simulink model "eulerEq"  (R2023b)
settings: Solver=ode4  StartTime=0.0  StopTime=30000  FixedStep=0.01  RelTol=1e-3
values from neighbouring files (symbols this model uses):
  date = [2023, 1, 21, 13, 52, 0]    [main.m]    (also in main_nonLin.m)
  euler0 = [0; 0; 0]    [main.m]    (also in main_nonLin.m)
  w0 = h0./sat.I'    [main.m]    (also in main_nonLin.m)
undefined symbols (not defined in the file or in its folder): airDensity, astroConstants, control, DiscIntNeverNeededParam, ea0, earth, gyroscope, magneticConstants, magnetorquer, magSensor, orbit, physicsConstants, rw, sat, sunSensor
libraries: simulink x21, matrix_library x7, sharedtransform x5, dspindex x5, sharedutil x4, vrlib x3, dspfactors x1, simulink_extras x1
(part 1 of 2)
settings Model: PauseTimes=3000  SnapshotBufferSize=100  SnapshotInterval=1  Creator=tomis  LastModifiedBy=francescoantoniomiccoli
settings SolverCC: AlgebraicLoopSolver=TrustRegion
settings DebuggingCC: UnconnectedInputMsg=warning  UnconnectedOutputMsg=warning  UnconnectedLineMsg=warning
settings ModelReferenceCC: EnableRefExpFcnMdlSchedulingChecks=on

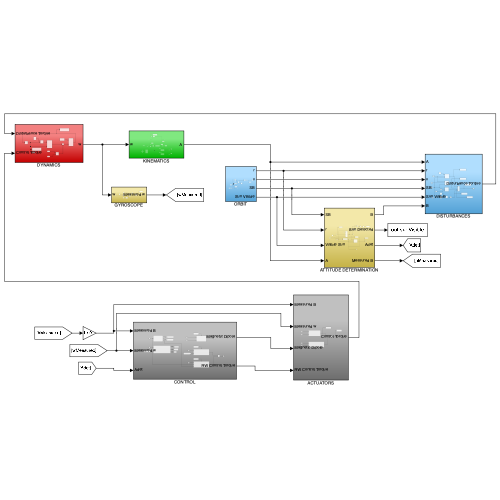
[thumbnail: Simulink's stored preview of the top-level diagram]
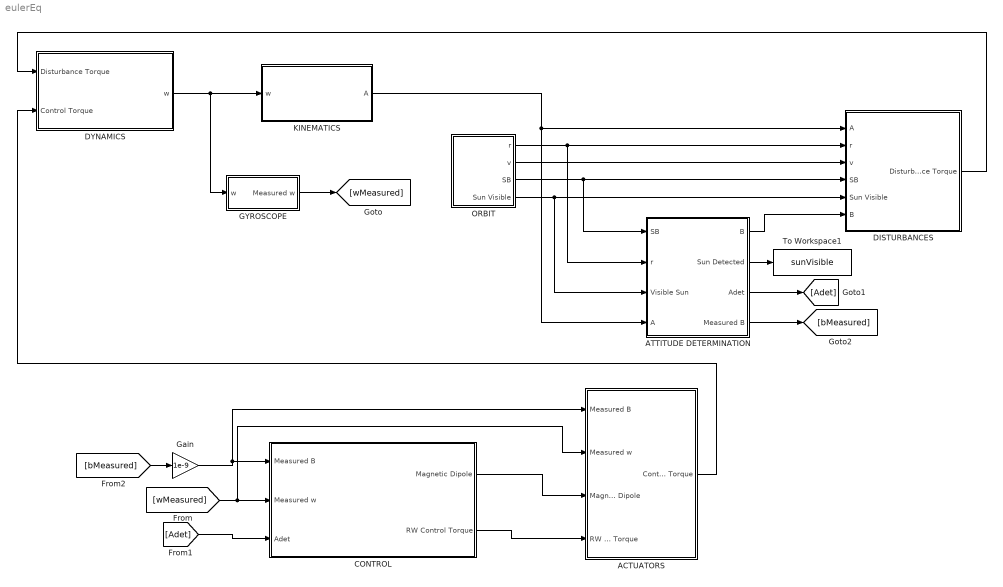
== system eulerEq ==
  ACTUATORS : Subsystem
  ATTITUDE DETERMINATION : Subsystem
  CONTROL : Subsystem
  DISTURBANCES : Subsystem
  DYNAMICS : Subsystem
  GYROSCOPE : Subsystem
  Gain : Gain  Gain=1e-9
  KINEMATICS : Subsystem
  ORBIT : Subsystem
  To Workspace1 : ToWorkspace  VariableName=sunVisible  SampleTime=-1
  wires:
  DYNAMICS/1(w) -> GYROSCOPE/1(w), KINEMATICS/1(w)
  KINEMATICS/1(A) -> DISTURBANCES/1(A), ATTITUDE DETERMINATION/4(A)
  ORBIT/1(r) -> ATTITUDE DETERMINATION/2(r), DISTURBANCES/2(r)
  ORBIT/2(v) -> DISTURBANCES/3(v)
  ORBIT/3(SB) -> ATTITUDE DETERMINATION/1(SB), DISTURBANCES/4(SB)
  ORBIT/4(Sun Visible) -> ATTITUDE DETERMINATION/3(Visible Sun), DISTURBANCES/5(Sun Visible)
  ATTITUDE DETERMINATION/1(B) -> DISTURBANCES/6(B)
  [wMeasured] -> CONTROL/2(Measured w), ACTUATORS/2(Measured w)
  [Adet] -> CONTROL/3(Adet)
  ATTITUDE DETERMINATION/4(Measured B) -> [bMeasured]
  [bMeasured] -> Gain/1
  CONTROL/1(Magnetic Dipole) -> ACTUATORS/3(Magnetic Dipole)
  CONTROL/2(RW Control Torque) -> ACTUATORS/4(RW Control Torque)
  Gain/1 -> CONTROL/1(Measured B), ACTUATORS/1(Measured B)
  DISTURBANCES/1(Disturbance Torque) -> DYNAMICS/1(Disturbance Torque)
  ATTITUDE DETERMINATION/2(Sun Detected) -> To Workspace1/1
  GYROSCOPE/1(Measured w) -> [wMeasured]
  ACTUATORS/1(Control Torque) -> DYNAMICS/2(Control Torque)
  ATTITUDE DETERMINATION/3(Adet) -> [Adet]

== system eulerEq/ACTUATORS ==
  Measured B : Inport
  Measured w : Inport  Port=2
  Magnetic Dipole : Inport  Port=3
  RW Control Torque : Inport  Port=4
  Add : Sum
  MAGNETORQUER : Subsystem
  REACTION WHEELS : Subsystem
  To Workspace : ToWorkspace  VariableName=controlTorque  SampleTime=-1
  To Workspace1 : ToWorkspace  VariableName=magneticTorque  SampleTime=-1
  Control Torque : Outport
  wires:
  Measured B/1 -> MAGNETORQUER/1(Measured B)
  Magnetic Dipole/1 -> MAGNETORQUER/2(Magnetic Dipole)
  MAGNETORQUER/1(Out1) -> To Workspace1/1, Add/1
  Add/1 -> To Workspace/1, Control Torque/1
  Measured w/1 -> REACTION WHEELS/2(Measured w)
  REACTION WHEELS/1(Out1) -> Add/2
  RW Control Torque/1 -> REACTION WHEELS/1(RW Control Torque)

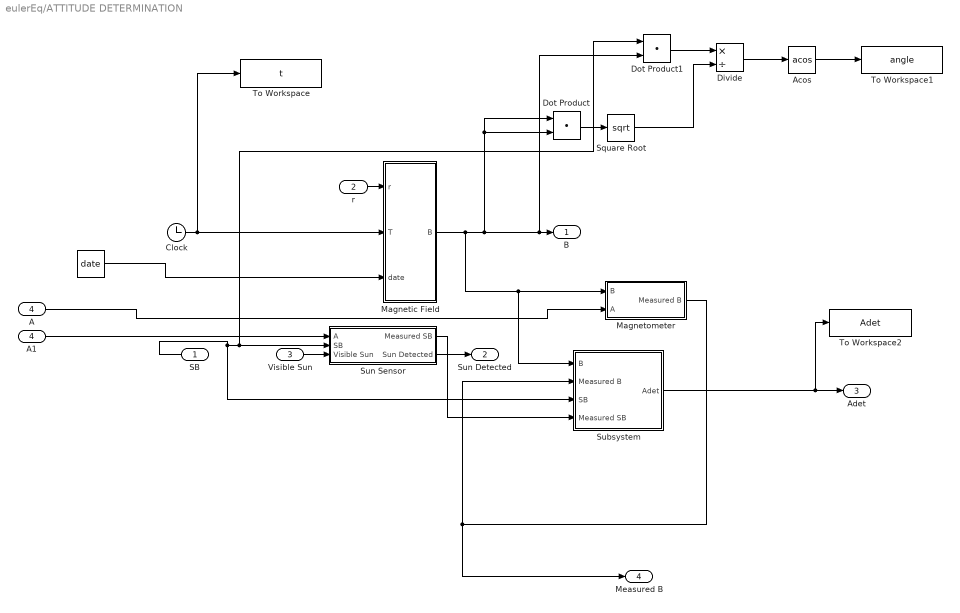
== system eulerEq/ATTITUDE DETERMINATION ==
  SB : Inport
  r : Inport  Port=2
  Visible Sun : Inport  Port=3
  A : Inport  Port=4
  " " : Constant  Value=date  VectorParams1D=off
  A1 : InportShadow  Port=4
  Acos : Trigonometry  Operator=acos
  Clock : Clock
  Divide : Product  Inputs=*/
  Dot Product : DotProduct  OutDataTypeStr=Inherit: Inherit via internal rule
  Dot Product1 : DotProduct  OutDataTypeStr=Inherit: Inherit via internal rule
  Magnetic Field : Subsystem
  Magnetometer : Subsystem
  Square Root : Sqrt
  Subsystem : Subsystem
  Sun Sensor : Subsystem
  To Workspace : ToWorkspace  VariableName=t  SampleTime=-1
  To Workspace1 : ToWorkspace  VariableName=angle  SampleTime=-1
  To Workspace2 : ToWorkspace  VariableName=Adet  SampleTime=-1
  B : Outport
  Sun Detected : Outport  Port=2
  Adet : Outport  Port=3
  Measured B : Outport  Port=4
  wires:
  Sun Sensor/2(Sun Detected) -> Sun Detected/1
  r/1 -> Magnetic Field/1(r)
  " "/1 -> Magnetic Field/3(date)
  Magnetic Field/1(B) -> Dot Product1/2, B/1, Dot Product/1, Dot Product/2, Subsystem/1(B), Magnetometer/1(B)
  Clock/1 -> To Workspace/1, Magnetic Field/2(T)
  Magnetometer/1(Measured B) -> Measured B/1, Subsystem/2(Measured B)
  A1/1 -> Sun Sensor/1(A)
  Subsystem/1(Adet) -> To Workspace2/1, Adet/1
  A/1 -> Magnetometer/2(A)
  Visible Sun/1 -> Sun Sensor/3(Visible Sun)
  SB/1 -> Subsystem/3(SB), Dot Product1/1, Sun Sensor/2(SB)
  Dot Product/1 -> Square Root/1
  Dot Product1/1 -> Divide/1
  Square Root/1 -> Divide/2
  Divide/1 -> Acos/1
  Acos/1 -> To Workspace1/1
  Sun Sensor/1(Measured SB) -> Subsystem/4(Measured SB)

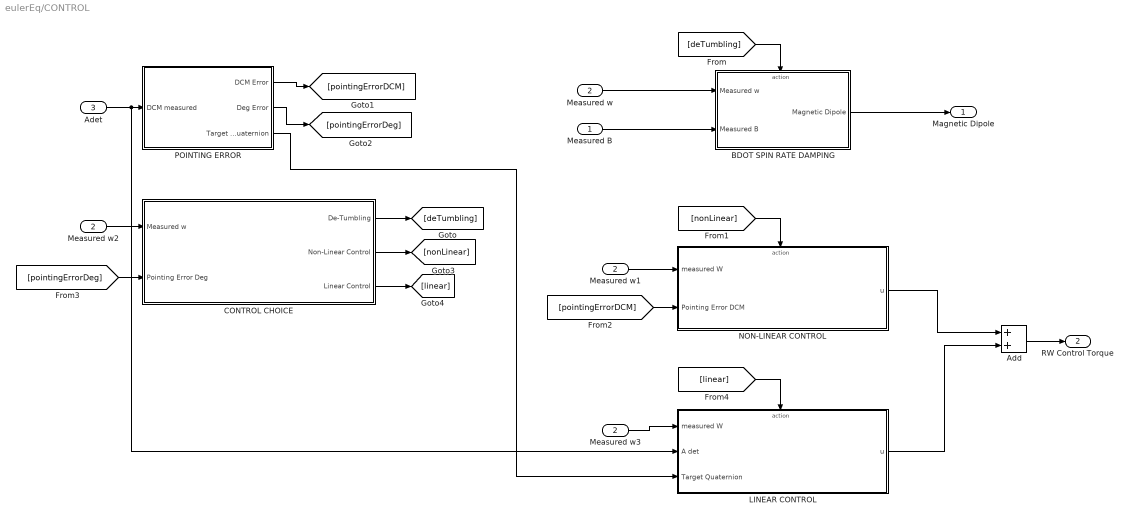
== system eulerEq/CONTROL ==
  Measured B : Inport
  Measured w : Inport  Port=2
  Adet : Inport  Port=3
  Add : Sum
  "BDOT SPIN RATE DAMPING " : Subsystem
  CONTROL CHOICE : Subsystem
  LINEAR CONTROL : Subsystem
  Measured w1 : InportShadow  Port=2
  Measured w2 : InportShadow  Port=2
  Measured w3 : InportShadow  Port=2
  NON-LINEAR CONTROL : Subsystem
  POINTING ERROR : Subsystem
  Magnetic Dipole : Outport
  RW Control Torque : Outport  Port=2
  wires:
  Measured B/1 -> "BDOT SPIN RATE DAMPING "/2(Measured B)
  [linear] -> LINEAR CONTROL/Action
  [nonLinear] -> NON-LINEAR CONTROL/Action
  Measured w2/1 -> CONTROL CHOICE/1(Measured w)
  CONTROL CHOICE/3(Linear Control) -> [linear]
  Add/1 -> RW Control Torque/1
  [pointingErrorDCM] -> NON-LINEAR CONTROL/2(Pointing Error DCM)
  NON-LINEAR CONTROL/1(u) -> Add/1
  Measured w1/1 -> NON-LINEAR CONTROL/1(measured W)
  Measured w/1 -> "BDOT SPIN RATE DAMPING "/1(Measured w)
  [deTumbling] -> "BDOT SPIN RATE DAMPING "/Action
  CONTROL CHOICE/1(De-Tumbling) -> [deTumbling]
  Adet/1 -> LINEAR CONTROL/2(A det), POINTING ERROR/1(DCM measured)
  POINTING ERROR/1(DCM Error) -> [pointingErrorDCM]
  POINTING ERROR/2(Deg Error) -> [pointingErrorDeg]
  [pointingErrorDeg] -> CONTROL CHOICE/2("Pointing Error Deg ")
  LINEAR CONTROL/1(u) -> Add/2
  "BDOT SPIN RATE DAMPING "/1(Magnetic Dipole) -> Magnetic Dipole/1
  CONTROL CHOICE/2(Non-Linear Control) -> [nonLinear]
  Measured w3/1 -> LINEAR CONTROL/1(measured W)
  POINTING ERROR/3(Target Quaternion) -> LINEAR CONTROL/3(Target Quaternion)

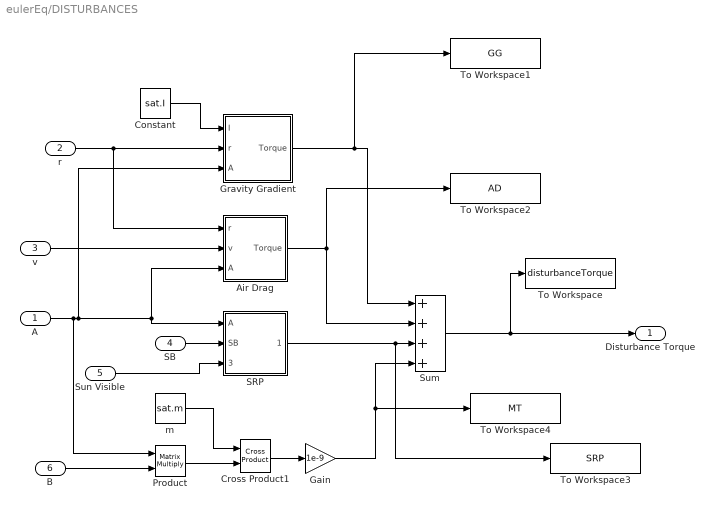
== system eulerEq/DISTURBANCES ==
  A : Inport
  r : Inport  Port=2
  v : Inport  Port=3
  SB : Inport  Port=4
  Sun Visible : Inport  Port=5
  B : Inport  Port=6
  Air Drag : Subsystem
  Constant : Constant  Value=sat.I
  Cross Product1 : vrlib/Utilities/Cross Product
  Gain : Gain  Gain=1e-9
  Gravity Gradient : Subsystem
  Product : Product  Multiplication=Matrix(*)
  SRP : Subsystem
  Sum : Sum  Inputs=++++
  To Workspace : ToWorkspace  VariableName=disturbanceTorque  SampleTime=-1
  To Workspace1 : ToWorkspace  VariableName=GG  SampleTime=-1
  To Workspace2 : ToWorkspace  VariableName=AD  SampleTime=-1
  To Workspace3 : ToWorkspace  VariableName=SRP  SampleTime=-1
  To Workspace4 : ToWorkspace  VariableName=MT  SampleTime=-1
  m : Constant  Value=sat.m
  Disturbance Torque : Outport
  wires:
  A/1 -> Product/1, Gravity Gradient/3(A), Air Drag/3(A), SRP/1(A)
  Sum/1 -> To Workspace/1, Disturbance Torque/1
  Constant/1 -> Gravity Gradient/1(I)
  r/1 -> Air Drag/1(r), Gravity Gradient/2(r)
  v/1 -> Air Drag/2(v)
  SB/1 -> SRP/2(SB)
  m/1 -> Cross Product1/1
  Cross Product1/1 -> Gain/1
  Sun Visible/1 -> SRP/3(Sun Visible)
  Product/1 -> Cross Product1/2
  B/1 -> Product/2
  Gravity Gradient/1(Torque) -> To Workspace1/1, Sum/1
  Air Drag/1(Torque) -> To Workspace2/1, Sum/2
  SRP/1(Torque) -> To Workspace3/1, Sum/3
  Gain/1 -> Sum/4, To Workspace4/1

== system eulerEq/DYNAMICS ==
  Disturbance Torque : Inport
  Control Torque : Inport  Port=2
  Add : Sum
  Constant : Constant  Value=diag(sat.I)
  Constant1 : Constant  Value=inv(diag(sat.I))
  Cross Product : matrix_library/Cross Product
  Integrator : Integrator  InitialCondition=w0
  Product : Product  Multiplication=Matrix(*)
  Product2 : Product  Multiplication=Matrix(*)
  Sum : Sum  Inputs=|++
  To Workspace : ToWorkspace  VariableName=w  SampleTime=-1
  To Workspace1 : ToWorkspace  VariableName=dw  SampleTime=-1
  w : Outport
  wires:
  Disturbance Torque/1 -> Add/1
  Control Torque/1 -> Add/2
  Constant1/1 -> Product/1
  Product/1 -> To Workspace1/1, Integrator/1
  Constant/1 -> Product2/1
  Integrator/1 -> w/1, To Workspace/1, Cross Product/2, Product2/2
  Product2/1 -> Cross Product/1
  Cross Product/1 -> Sum/1
  Add/1 -> Sum/2
  Sum/1 -> Product/2

== system eulerEq/GYROSCOPE ==
  w : Inport
  ARW : RandomNumber  Variance=gyroscope.stdDeviation^2  Seed=12984537  SampleTime=gyroscope.Ts  VectorParams1D=off
  Add : Sum  Inputs=+++
  Discrete-Time Integrator : DiscreteIntegrator  IntegratorMethod=Integration: Trapezoidal  SampleTime=gyroscope.Ts  ICPrevOutput=DiscIntNeverNeededParam  ICPrevScaledInput=DiscIntNeverNeededParam
  MatrixMultiply : Product  Multiplication=Matrix(*)
  MatrixMultiply1 : Product  Multiplication=Matrix(*)
  RRW : RandomNumber  Variance=gyroscope.biasStability^2  Seed=34654365  SampleTime=gyroscope.Ts  VectorParams1D=off
  Rotation B-S : Constant  Value=eye(3)
  Rotation S-B : Constant  Value=eye(3)
  To Workspace5 : ToWorkspace  VariableName=wdet  SampleTime=-1
  Measured w : Outport
  wires:
  Add/1 -> MatrixMultiply1/2
  Rotation S-B/1 -> MatrixMultiply1/1
  Discrete-Time Integrator/1 -> Add/3
  MatrixMultiply/1 -> Add/2
  w/1 -> MatrixMultiply/2
  Rotation B-S/1 -> MatrixMultiply/1
  ARW/1 -> Add/1
  RRW/1 -> Discrete-Time Integrator/1
  MatrixMultiply1/1 -> To Workspace5/1, Measured w/1

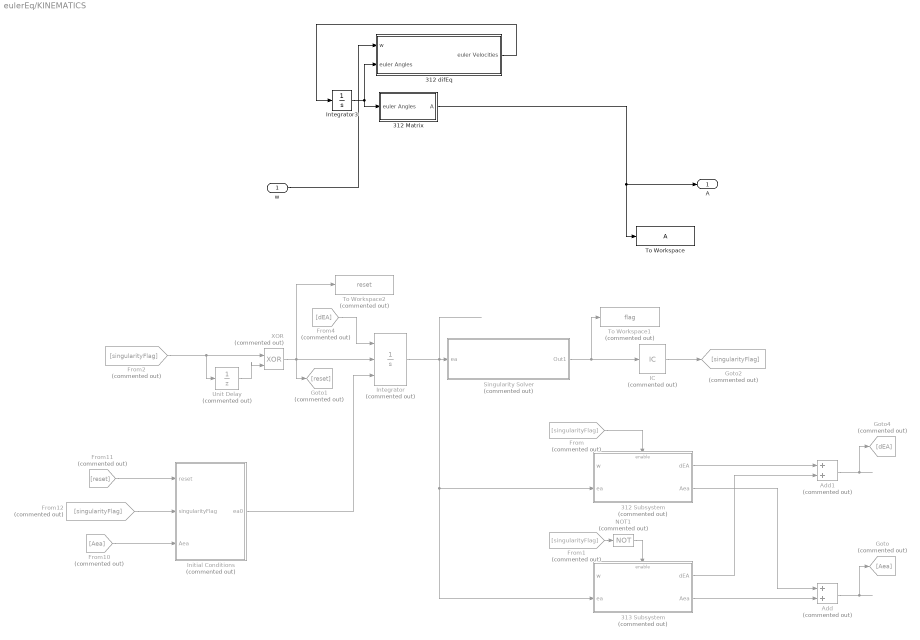
== system eulerEq/KINEMATICS ==
  w : Inport
  312 Matrix : Subsystem
  312 Subsystem : Subsystem  Commented=on  TreatAsAtomicUnit=on
  312 difEq : Subsystem
  313 Subsystem : Subsystem  Commented=on  TreatAsAtomicUnit=on
  Add : Sum  Commented=on
  Add1 : Sum  Commented=on
  From{,1..2,12} (4 alike) : From  Commented=on  GotoTag=singularityFlag
  From10 : From  Commented=on  GotoTag=Aea
  From11 : From  Commented=on  GotoTag=reset
  From4 : From  Commented=on  GotoTag=dEA
  Goto : Goto  Commented=on  GotoTag=Aea
  Goto1 : Goto  Commented=on  GotoTag=reset
  Goto2 : Goto  Commented=on  GotoTag=singularityFlag
  Goto4 : Goto  Commented=on  GotoTag=dEA
  IC : InitialCondition  Commented=on
  Initial Conditions : Subsystem  Commented=on
  Integrator : Integrator  Commented=on  ExternalReset=rising  InitialConditionSource=external
  Integrator3 : Integrator  InitialCondition=euler0
  NOT1 : Logic  Commented=on  Operator=NOT  AllPortsSameDT=off  OutDataTypeStr=boolean
  Singularity Solver : Subsystem  Commented=on
  To Workspace : ToWorkspace  VariableName=A  SampleTime=-1
  To Workspace1 : ToWorkspace  Commented=on  VariableName=flag  SampleTime=-1
  To Workspace2 : ToWorkspace  Commented=on  VariableName=reset  SampleTime=-1
  Unit Delay : UnitDelay  Commented=on  InitialCondition=1  SampleTime=-1  HasFrameUpgradeWarning=on
  XOR : Logic  Commented=on  Operator=XOR  IconShape=distinctive  AllPortsSameDT=off  OutDataTypeStr=boolean
  A : Outport
  wires:
  312 difEq/1(euler Velocities) -> Integrator3/1
  Integrator3/1 -> 312 Matrix/1(euler Angles), 312 difEq/2(euler Angles)
  w/1 -> 312 difEq/1(w)
  312 Matrix/1(A) -> To Workspace/1, A/1
  Singularity Solver/1(Out1) -> IC/1, To Workspace1/1
  312 Subsystem/2(Aea) -> Add/1
  313 Subsystem/1(dEA) -> Add1/2
  312 Subsystem/1(dEA) -> Add1/1
  Integrator/1 -> 313 Subsystem/2(ea), 312 Subsystem/2(ea), Singularity Solver/1(ea)
  Add1/1 -> Goto4/1
  IC/1 -> Goto2/1
  From10/1 -> Initial Conditions/3(Aea)
  From1/1 -> NOT1/1
  XOR/1 -> To Workspace2/1, Integrator/2, Goto1/1
  313 Subsystem/2(Aea) -> Add/2
  From4/1 -> Integrator/1
  From12/1 -> Initial Conditions/2(singularityFlag)
  From2/1 -> Unit Delay/1, XOR/1
  From11/1 -> Initial Conditions/1(reset)
  From/1 -> 312 Subsystem/Enable
  Unit Delay/1 -> XOR/2
  Add/1 -> Goto/1
  NOT1/1 -> 313 Subsystem/Enable
  Initial Conditions/1(ea0) -> Integrator/3

== system eulerEq/ORBIT ==
  Cross Product : matrix_library/Cross Product
  Cross Product1 : matrix_library/Cross Product
  Earth Orbit : Subsystem
  Gain2 : Gain  Gain=-1
  Matrix Concatenate : Concatenate  NumInputs=3  Mode=Multidimensional array  ConcatenateDimension=2
  Normalize1 : Subsystem
  Normalize2 : Subsystem
  Normalize3 : Subsystem
  Sat Orbit : Subsystem
  Sun Detection : Subsystem
  To Workspace : ToWorkspace  VariableName=DCMTarget  SampleTime=-1
  To Workspace1 : ToWorkspace  VariableName=rorbit  SampleTime=-1
  Transpose : Math  Operator=transpose
  r : Outport
  v : Outport  Port=2
  SB : Outport  Port=3
  Sun Visible : Outport  Port=4
  tag scope: DCMTarget=global
  wires:
  Sat Orbit/1(r) -> Sun Detection/1(r), Normalize2/1(r), To Workspace1/1, r/1
  Earth Orbit/1(r) -> Normalize1/1(r)
  Normalize1/1(Out) -> Gain2/1
  Sat Orbit/2(v) -> Normalize3/1(r), v/1
  Gain2/1 -> Sun Detection/2(SB), SB/1
  Sun Detection/1(Sun Visible) -> Sun Visible/1
  Normalize2/1(Out) -> Cross Product1/2, Matrix Concatenate/3, Cross Product/1
  Normalize3/1(Out) -> Cross Product/2
  Cross Product/1 -> Matrix Concatenate/2, Cross Product1/1
  Cross Product1/1 -> Matrix Concatenate/1
  Matrix Concatenate/1 -> Transpose/1
  Transpose/1 -> To Workspace/1, [DCMTarget]

== system eulerEq/ACTUATORS/MAGNETORQUER ==
  Measured B : Inport
  Magnetic Dipole : Inport  Port=2
  Cross Product : matrix_library/Cross Product
  Saturation : Saturate  UpperLimit=magnetorquer.m  LowerLimit=-magnetorquer.m
  To Workspace : ToWorkspace  VariableName=dipole  SampleTime=-1
  Out1 : Outport
  wires:
  Magnetic Dipole/1 -> Saturation/1
  Measured B/1 -> Cross Product/2
  Cross Product/1 -> Out1/1
  Saturation/1 -> To Workspace/1, Cross Product/1

== system eulerEq/ACTUATORS/REACTION WHEELS ==
  RW Control Torque : Inport
  Measured w : Inport  Port=2
  Add : Sum
  Add1 : Sum
  Constant : Constant  Value=rw.Ainv
  Constant1 : Constant  Value=rw.A
  Cross Product : matrix_library/Cross Product
  Gain : Gain  Gain=-1
  Gain1 : Gain  Gain=-1
  Integrator : Integrator
  Product : Product  Multiplication=Matrix(*)
  Product1 : Product  Multiplication=Matrix(*)
  Product2 : Product  Multiplication=Matrix(*)
  Saturation : Saturate  UpperLimit=rw.dhMax  LowerLimit=-rw.dhMax
  Saturation1 : Saturate  UpperLimit=rw.hMax  LowerLimit=-rw.hMax
  To Workspace : ToWorkspace  VariableName=hr  SampleTime=-1
  To Workspace1 : ToWorkspace  VariableName=dhr  SampleTime=-1
  Out1 : Outport
  wires:
  Constant/1 -> Gain/1
  Gain/1 -> Product/1
  Measured w/1 -> Cross Product/1
  Product1/1 -> Cross Product/2
  Constant1/1 -> Product1/1, Product2/1
  Cross Product/1 -> Add1/1, Add/2
  Add/1 -> Product/2
  RW Control Torque/1 -> Add/1
  Product/1 -> Saturation/1
  Product2/1 -> Add1/2
  Add1/1 -> Gain1/1
  Gain1/1 -> Out1/1
  Integrator/1 -> Saturation1/1
  Saturation/1 -> To Workspace1/1, Integrator/1, Product2/2
  Saturation1/1 -> To Workspace/1, Product1/2

== system eulerEq/ATTITUDE DETERMINATION/Magnetic Field ==
  r : Inport
  T : Inport  Port=2
  date : Inport  Port=3
  MATLAB Function : MATLAB Function  TreatAsAtomicUnit=on
  Transpose : Math  Operator=transpose
  igrfSg : Constant  Value=magneticConstants.igrfSg
  igrfSh : Constant  Value=magneticConstants.igrfSh
  B : Outport
  wires:
  igrfSh/1 -> MATLAB Function/5(igrfSh)
  T/1 -> MATLAB Function/2(T)
  igrfSg/1 -> MATLAB Function/4(igrfSg)
  r/1 -> Transpose/1
  date/1 -> MATLAB Function/3(date)
  Transpose/1 -> MATLAB Function/1(r)
  MATLAB Function/1(B) -> B/1

== system eulerEq/ATTITUDE DETERMINATION/Magnetometer ==
  B : Inport
  A : Inport  Port=2
  Band-Limited White Noise : simulink/Sources/Band-Limited White Noise  Cov=magSensor.noisePower*[1;1;1]  Ts=1/magSensor.sampleRate  seed=[3563456;34634;7567457]  VectorParams1D=off
  Product : Product  Multiplication=Matrix(*)
  Quantizer : Quantizer  QuantizationInterval=magSensor.resolution
  Sum : Sum  Inputs=|++
  Zero-Order Hold : ZeroOrderHold  SampleTime=1/magSensor.sampleRate
  Measured B : Outport
  wires:
  Zero-Order Hold/1 -> Sum/1
  Band-Limited White Noise/1 -> Sum/2
  Sum/1 -> Quantizer/1
  Quantizer/1 -> Measured B/1
  B/1 -> Product/2
  Product/1 -> Zero-Order Hold/1
  A/1 -> Product/1

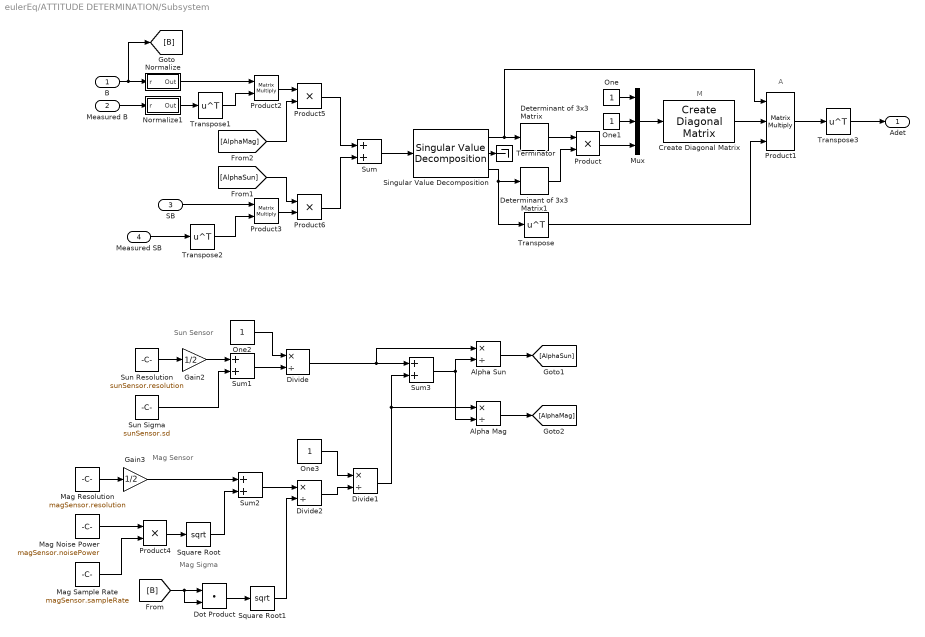
== system eulerEq/ATTITUDE DETERMINATION/Subsystem ==
  note: Mag Sigma
  note: Sun Sensor
  note: A
  note: M
  note: Mag Sensor
  B : Inport
  Measured B : Inport  Port=2
  SB : Inport  Port=3
  Measured SB : Inport  Port=4
  Alpha Mag : Product  Inputs=*/
  Alpha Sun : Product  Inputs=*/
  Create Diagonal Matrix : matrix_library/Create Diagonal Matrix
      settings: LibrarySourceBlock=|
      | simulink/Matrix
      | Operations/Create Diagonal
      | Matrix
  Determinant of 3x3 Matrix : sharedutil/Determinant of 3x3 Matrix  aMode=aMode
      settings: LibrarySourceBlock=|
      | aerolibutil/Determinant of
      | 3x3 Matrix
  Determinant of 3x3 Matrix1 : sharedutil/Determinant of 3x3 Matrix  aMode=aMode
      settings: LibrarySourceBlock=|
      | aerolibutil/Determinant of
      | 3x3 Matrix
  Divide : Product  Inputs=*/
  Divide1 : Product  Inputs=*/
  Divide2 : Product  Inputs=*/
  Dot Product : DotProduct  OutDataTypeStr=Inherit: Inherit via internal rule
  Gain2 : Gain  Gain=1/2
  Gain3 : Gain  Gain=1/2
  Mag Noise Power : Constant  Value=magSensor.noisePower
  Mag Resolution : Constant  Value=magSensor.resolution
  Mag Sample Rate : Constant  Value=magSensor.sampleRate
  Mux : Mux  Inputs=3
  Normalize : Subsystem
  Normalize1 : Subsystem
  One{,1..3} (4 alike) : Constant  OutDataTypeStr=Inherit: Inherit via back propagation
  Product{,4..6} (4 alike) : Product
  Product1 : Product  Inputs=3  Multiplication=Matrix(*)
  Product2 : Product  Multiplication=Matrix(*)
  Product3 : Product  Multiplication=Matrix(*)
  Singular Value Decomposition : dspfactors/Singular Value Decomposition  wantv=on  wanterr=off  SimulateUsing=Interpreted execution
  Square Root : Sqrt
  Square Root1 : Sqrt
  Sum{,1..3} (4 alike) : Sum
  Sun Resolution : Constant  Value=sunSensor.resolution
  Sun Sigma : Constant  Value=sunSensor.sd
  Terminator : Terminator
  Transpose{,1..3} (4 alike) : Math  Operator=transpose
  Adet : Outport
  wires:
  Sum/1 -> Singular Value Decomposition/1
  One/1 -> Mux/1
  Normalize1/1(Out) -> Transpose1/1
  Singular Value Decomposition/1 -> Determinant of 3x3 Matrix/1, Product1/1
  Create Diagonal Matrix/1 -> Product1/2
  Transpose/1 -> Product1/3
  Singular Value Decomposition/3 -> Transpose/1, Determinant of 3x3 Matrix1/1
  One1/1 -> Mux/2
  Transpose2/1 -> Product3/2
  Determinant of 3x3 Matrix/1 -> Product/1
  Measured B/1 -> Normalize1/1(r)
  Singular Value Decomposition/2 -> Terminator/1
  Determinant of 3x3 Matrix1/1 -> Product/2
  Mux/1 -> Create Diagonal Matrix/1
  Product/1 -> Mux/3
  Transpose1/1 -> Product2/2
  Product1/1 -> Transpose3/1
  Normalize/1(Out) -> Product2/1
  B/1 -> [B], Normalize/1(r)
  SB/1 -> Product3/1
  Measured SB/1 -> Transpose2/1
  Sun Resolution/1 -> Gain2/1
  Gain2/1 -> Sum1/1
  Sun Sigma/1 -> Sum1/2
  Sum1/1 -> Divide/2
  One2/1 -> Divide/1
  Mag Noise Power/1 -> Product4/1
  Mag Sample Rate/1 -> Product4/2
  Product4/1 -> Square Root/1
  Mag Resolution/1 -> Gain3/1
  Gain3/1 -> Sum2/1
  Square Root/1 -> Sum2/2
  One3/1 -> Divide1/1
  Divide/1 -> Alpha Sun/1, Sum3/1
  Divide1/1 -> Sum3/2, Alpha Mag/1
  Sum3/1 -> Alpha Mag/2, Alpha Sun/2
  Sum2/1 -> Divide2/1
  Divide2/1 -> Divide1/2
  Product2/1 -> Product5/1
  Product3/1 -> Product6/2
  Alpha Sun/1 -> [AlphaSun]
  Alpha Mag/1 -> [AlphaMag]
  [AlphaSun] -> Product6/1
  [AlphaMag] -> Product5/2
  Product5/1 -> Sum/1
  Product6/1 -> Sum/2
  [B] -> Dot Product/2, Dot Product/1
  Dot Product/1 -> Square Root1/1
  Square Root1/1 -> Divide2/2
  Transpose3/1 -> Adet/1

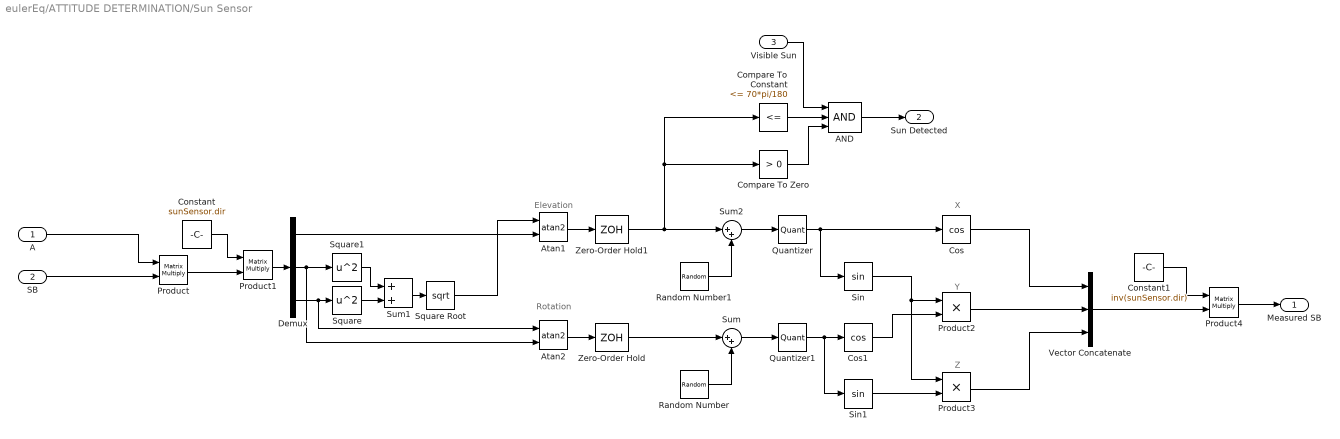
== system eulerEq/ATTITUDE DETERMINATION/Sun Sensor ==
  note: Y
  note: Z
  note: X
  note: Rotation
  note: Elevation
  A : Inport
  SB : Inport  Port=2
  Visible Sun : Inport  Port=3
  AND : Logic  Inputs=3  IconShape=distinctive  AllPortsSameDT=off  OutDataTypeStr=boolean
  Atan1 : Trigonometry  Operator=atan2
  Atan2 : Trigonometry  Operator=atan2
  Compare To Constant : simulink/Logic and Bit Operations/Compare To Constant  relop=<=  const=70*pi/180  OutDataTypeStr=boolean
  Compare To Zero : simulink/Logic and Bit Operations/Compare To Zero  relop=>  OutDataTypeStr=boolean
  Constant : Constant  Value=sunSensor.dir
  Constant1 : Constant  Value=inv(sunSensor.dir)
  Cos : Trigonometry  Operator=cos
  Cos1 : Trigonometry  Operator=cos
  Demux : Demux  Outputs=3
  Product : Product  Multiplication=Matrix(*)
  Product1 : Product  Multiplication=Matrix(*)
  Product2 : Product
  Product3 : Product
  Product4 : Product  Multiplication=Matrix(*)
  Quantizer : Quantizer  QuantizationInterval=sunSensor.resolution
  Quantizer1 : Quantizer  QuantizationInterval=sunSensor.resolution
  Random Number : RandomNumber  Variance=sunSensor.sd^2  Seed=76538356  SampleTime=1/sunSensor.sampleRate
  Random Number1 : RandomNumber  Variance=sunSensor.sd^2  Seed=45746823  SampleTime=1/sunSensor.sampleRate
  Sin : Trigonometry
  Sin1 : Trigonometry
  Square : Math  Operator=square
  Square Root : Sqrt
  Square1 : Math  Operator=square
  Sum : Sum  Inputs=|++
  Sum1 : Sum
  Sum2 : Sum  Inputs=|++
  Vector Concatenate : Concatenate  NumInputs=3  ConcatenateDimension=2
  Zero-Order Hold : ZeroOrderHold  SampleTime=1/sunSensor.sampleRate
  Zero-Order Hold1 : ZeroOrderHold  SampleTime=1/sunSensor.sampleRate
  Measured SB : Outport
  Sun Detected : Outport  Port=2
  wires:
  Cos1/1 -> Product2/2
  Square/1 -> Sum1/2
  Zero-Order Hold/1 -> Sum/1
  Square1/1 -> Sum1/1
  Random Number/1 -> Sum/2
  Sum2/1 -> Quantizer/1
  Product/1 -> Product1/2
  Sin/1 -> Product3/1, Product2/1
  Constant/1 -> Product1/1
  Demux/2 -> Square1/1, Atan2/2
  Demux/3 -> Atan2/1, Square/1
  Sin1/1 -> Product3/2
  Atan2/1 -> Zero-Order Hold/1
  Atan1/1 -> Zero-Order Hold1/1
  Product1/1 -> Demux/1
  Sum1/1 -> Square Root/1
  Quantizer1/1 -> Sin1/1, Cos1/1
  Zero-Order Hold1/1 -> Compare To Zero/1, Compare To Constant/1, Sum2/1
  Product2/1 -> Vector Concatenate/2
  Sum/1 -> Quantizer1/1
  A/1 -> Product/1
  SB/1 -> Product/2
  Product3/1 -> Vector Concatenate/3
  Quantizer/1 -> Sin/1, Cos/1
  Cos/1 -> Vector Concatenate/1
  Vector Concatenate/1 -> Product4/2
  Constant1/1 -> Product4/1
  Product4/1 -> Measured SB/1
  Random Number1/1 -> Sum2/2
  Compare To Constant/1 -> AND/2
  Visible Sun/1 -> AND/1
  AND/1 -> Sun Detected/1
  Compare To Zero/1 -> AND/3
  Demux/1 -> Atan1/2
  Square Root/1 -> Atan1/1

== system eulerEq/CONTROL/BDOT SPIN RATE DAMPING  ==
  Measured w : Inport
  Measured B : Inport  Port=2
  Action Port : ActionPort  ActionPortLabel=else
  CROSS MATRIX : Subsystem
  Constant : Constant  Value=-5e7
  Gain : Gain  Gain=-1
  Product : Product  Multiplication=Matrix(*)
  Product1 : Product
  Magnetic Dipole : Outport  OutputWhenDisabled=reset  InitialOutput=[0;0;0]
  wires:
  Measured w/1 -> CROSS MATRIX/1(Measured w)
  CROSS MATRIX/1(w^) -> Gain/1
  Gain/1 -> Product/1
  Measured B/1 -> Product/2
  Product/1 -> Product1/2  "dB"
  Product1/1 -> Magnetic Dipole/1
  Constant/1 -> Product1/1

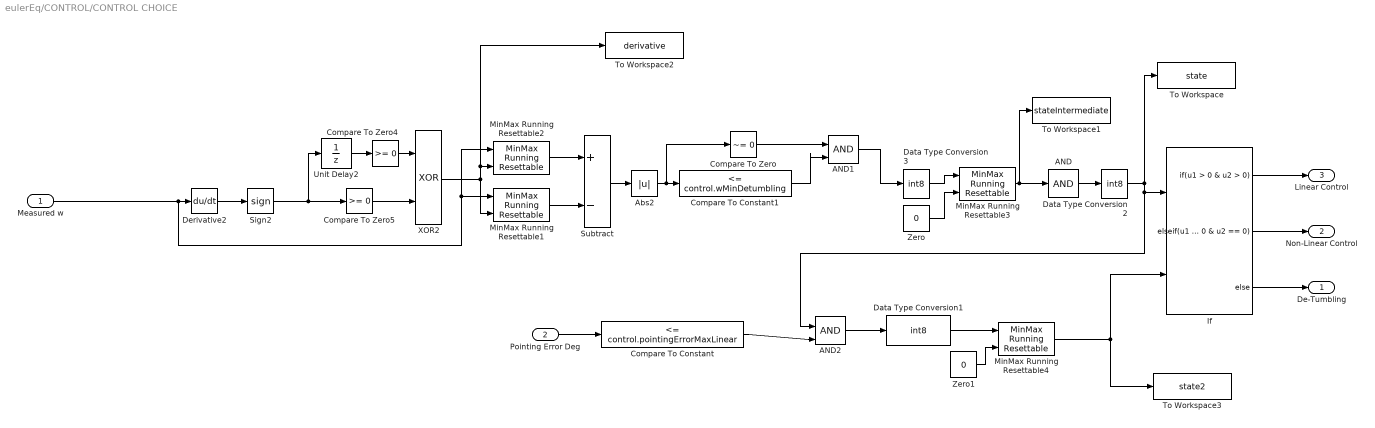
== system eulerEq/CONTROL/CONTROL CHOICE ==
  Measured w : Inport
  "Pointing Error Deg " : Inport  Port=2
  AND : Logic  Inputs=1  IconShape=distinctive  AllPortsSameDT=off  OutDataTypeStr=boolean
  AND1 : Logic  IconShape=distinctive  AllPortsSameDT=off  OutDataTypeStr=boolean
  AND2 : Logic  IconShape=distinctive  AllPortsSameDT=off  OutDataTypeStr=boolean
  Abs2 : Abs  SaturateOnIntegerOverflow=off
  Compare To Constant : simulink/Logic and Bit Operations/Compare To Constant  relop=<=  const=control.pointingErrorMaxLinear  OutDataTypeStr=boolean
  Compare To Constant1 : simulink/Logic and Bit Operations/Compare To Constant  relop=<=  const=control.wMinDetumbling  OutDataTypeStr=boolean
  Compare To Zero : simulink/Logic and Bit Operations/Compare To Zero  relop=~=  OutDataTypeStr=boolean
  Compare To Zero4 : simulink/Logic and Bit Operations/Compare To Zero  relop=>=  OutDataTypeStr=boolean
  Compare To Zero5 : simulink/Logic and Bit Operations/Compare To Zero  relop=>=  OutDataTypeStr=boolean
  Data Type Conversion1 : DataTypeConversion  OutDataTypeStr=int8  SaturateOnIntegerOverflow=off  RndMeth=Floor
  Data Type Conversion2 : DataTypeConversion  OutDataTypeStr=int8  SaturateOnIntegerOverflow=off  RndMeth=Floor
  Data Type Conversion3 : DataTypeConversion  OutDataTypeStr=int8  SaturateOnIntegerOverflow=off  RndMeth=Floor
  Derivative2 : Derivative
  If : If  NumInputs=2  IfExpression=u1 > 0 & u2 > 0  ElseIfExpressions=u1 > 0 & u2 == 0
  MinMax Running Resettable1 : simulink/Math Operations/MinMax Running Resettable  Function=min  vinit=0.0
  MinMax Running Resettable2 : simulink/Math Operations/MinMax Running Resettable  Function=max  vinit=0
  MinMax Running Resettable3 : simulink/Math Operations/MinMax Running Resettable  Function=max  vinit=0
  MinMax Running Resettable4 : simulink/Math Operations/MinMax Running Resettable  Function=max  vinit=0
  Sign2 : Signum
  Subtract : Sum  Inputs=+-
  To Workspace : ToWorkspace  VariableName=state  SampleTime=-1
  To Workspace1 : ToWorkspace  VariableName=stateIntermediate  SampleTime=-1
  To Workspace2 : ToWorkspace  VariableName=derivative  SampleTime=-1
  To Workspace3 : ToWorkspace  VariableName=state2  SampleTime=-1
  Unit Delay2 : UnitDelay  InitialCondition=-1  SampleTime=-1  HasFrameUpgradeWarning=on
  XOR2 : Logic  Operator=XOR  AllPortsSameDT=off  OutDataTypeStr=boolean
  Zero : Constant  Value=0  OutDataTypeStr=Inherit: Inherit via back propagation
  Zero1 : Constant  Value=0  OutDataTypeStr=Inherit: Inherit via back propagation
  De-Tumbling : Outport
  Non-Linear Control : Outport  Port=2
  Linear Control : Outport  Port=3
  wires:
  Derivative2/1 -> Sign2/1
  Sign2/1 -> Unit Delay2/1, Compare To Zero5/1
  Compare To Zero5/1 -> XOR2/2
  Compare To Zero4/1 -> XOR2/1
  Unit Delay2/1 -> Compare To Zero4/1
  "Pointing Error Deg "/1 -> Compare To Constant/1
  If/1 -> Linear Control/1
  If/2 -> Non-Linear Control/1
  If/3 -> De-Tumbling/1
  XOR2/1 -> MinMax Running Resettable2/2, To Workspace2/1, MinMax Running Resettable1/2
  MinMax Running Resettable2/1 -> Subtract/1
  MinMax Running Resettable1/1 -> Subtract/2
  Abs2/1 -> Compare To Zero/1, Compare To Constant1/1
  Subtract/1 -> Abs2/1
  AND/1 -> Data Type Conversion2/1
  Data Type Conversion2/1 -> AND2/1, If/1, To Workspace/1
  MinMax Running Resettable3/1 -> To Workspace1/1, AND/1
  Data Type Conversion3/1 -> MinMax Running Resettable3/1
  Measured w/1 -> Derivative2/1, MinMax Running Resettable2/1, MinMax Running Resettable1/1
  Compare To Constant1/1 -> AND1/2
  AND1/1 -> Data Type Conversion3/1
  Compare To Zero/1 -> AND1/1
  Data Type Conversion1/1 -> MinMax Running Resettable4/1
  MinMax Running Resettable4/1 -> To Workspace3/1, If/2
  Zero/1 -> MinMax Running Resettable3/2
  Zero1/1 -> MinMax Running Resettable4/2
  AND2/1 -> Data Type Conversion1/1
  Compare To Constant/1 -> AND2/2

== system eulerEq/CONTROL/LINEAR CONTROL ==
  measured W : Inport
  A det : Inport  Port=2
  Target Quaternion : Inport  Port=3
  Action Port : ActionPort  ActionPortLabel=if(u1 > 0 & u2 > 0)
  Add : Sum  Inputs=-+
  Constant : Constant  Value=control.K
  Constant1 : Constant  Value=[control.wTarget]
  Direction Cosine Matrix to Quaternions : sharedtransform/Direction Cosine Matrix  to Quaternions  aMode=0  action=None  tolerance=eps(2)
      settings: LibrarySourceBlock=|
      | aerolibtransform2/Direction Cosine Matrix
      | to Quaternions
  Matrix Concatenate : Concatenate  Mode=Multidimensional array
  Product : Product  Multiplication=Matrix(*)
  Vector Concatenate : Concatenate
  u : Outport  OutputWhenDisabled=reset  InitialOutput=[0;0;0]
  wires:
  A det/1 -> Direction Cosine Matrix to Quaternions/1
  measured W/1 -> Vector Concatenate/1
  Constant/1 -> Product/1
  Direction Cosine Matrix to Quaternions/1 -> Vector Concatenate/2
  Vector Concatenate/1 -> Add/1
  Add/1 -> Product/2
  Product/1 -> u/1
  Constant1/1 -> Matrix Concatenate/1
  Target Quaternion/1 -> Matrix Concatenate/2
  Matrix Concatenate/1 -> Add/2

== system eulerEq/CONTROL/NON-LINEAR CONTROL ==
  measured W : Inport
  Pointing Error DCM : Inport  Port=2
  Action Port : ActionPort  ActionPortLabel=elseif(u1 > 0 & u2 == 0)
  Add1 : Sum
  Gain1 : Gain  Gain=-0.4
  Gain3 : Gain  Gain=-0.006
  u : Outport  OutputWhenDisabled=reset  InitialOutput=[0;0;0]
  wires:
  Add1/1 -> u/1
  Gain1/1 -> Add1/1
  measured W/1 -> Gain1/1
  Pointing Error DCM/1 -> Gain3/1
  Gain3/1 -> Add1/2

== system eulerEq/CONTROL/POINTING ERROR ==
  DCM measured : Inport
  Add : Sum  Inputs=+-
  Demux : Demux  Outputs=3
  Demux1 : Demux  Outputs=3
  Direction Cosine Matrix to Quaternions : sharedtransform/Direction Cosine Matrix  to Quaternions  aMode=0  action=None  tolerance=eps(2)
      settings: LibrarySourceBlock=|
      | aerolibtransform2/Direction Cosine Matrix
      | to Quaternions
  Gain : Gain  Gain=-1
  Gain1 : Gain  Gain=-1
  Multiport Selector : dspindex/Multiport Selector  rowsOrCols=Rows  idxCellArray={ 1,2 }  idxErrMode=Clip Index
      settings: LibrarySourceBlock=|
      | dsphdlsupportsigmgmt/Multiport
      | Selector
  Mux : Mux  Inputs=3
  POINTING ERROR (DEG) : Subsystem
  Product : Product  Multiplication=Matrix(*)
  Terminator : Terminator
  Terminator1 : Terminator
  Terminator2 : Terminator
  To Workspace : ToWorkspace  VariableName=degPointingError  SampleTime=-1
  Transpose : Math  Operator=transpose
  Transpose1 : Math  Operator=transpose
  DCM Error : Outport
  Deg Error : Outport  Port=2
  Target Quaternion : Outport  Port=3
  wires:
  [DCMTarget] -> Direction Cosine Matrix to Quaternions/1, Transpose/1
  Multiport Selector/1 -> Demux/1
  Multiport Selector/2 -> Demux1/1
  Gain/1 -> Mux/3
  Demux/2 -> Gain/1
  Demux/1 -> Terminator/1
  Demux/3 -> Mux/2
  Demux1/1 -> Terminator1/1
  Demux1/2 -> Terminator2/1
  Gain1/1 -> Mux/1
  Demux1/3 -> Gain1/1
  Transpose1/1 -> Add/1
  Mux/1 -> DCM Error/1
  Product/1 -> POINTING ERROR (DEG)/1(A * Ad^T), Add/2, Transpose1/1
  DCM measured/1 -> Product/1
  Transpose/1 -> Product/2
  Add/1 -> Multiport Selector/1
  POINTING ERROR (DEG)/1(Degrees out) -> To Workspace/1, Deg Error/1
  Direction Cosine Matrix to Quaternions/1 -> Target Quaternion/1

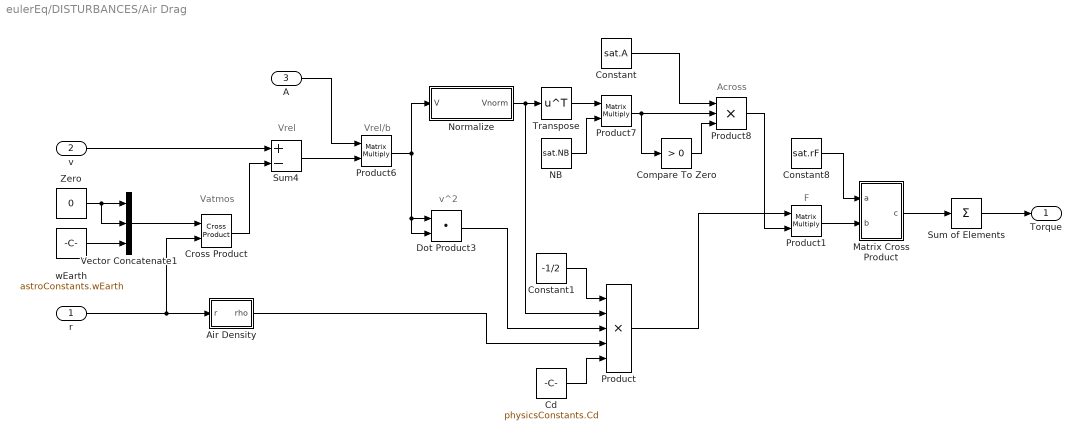
== system eulerEq/DISTURBANCES/Air Drag ==
  note: F
  note: v^2
  note: Across
  note: Vrel/b
  note: Vrel
  note: Vatmos
  r : Inport
  v : Inport  Port=2
  A : Inport  Port=3
  Air Density : Subsystem
  Cd : Constant  Value=physicsConstants.Cd
  Compare To Zero : simulink/Logic and Bit Operations/Compare To Zero  relop=>  OutDataTypeStr=boolean
  Constant : Constant  Value=sat.A
  Constant1 : Constant  Value=-1/2
  Constant8 : Constant  Value=sat.rF  VectorParams1D=off
  Cross Product : vrlib/Utilities/Cross Product
  Dot Product3 : DotProduct  OutDataTypeStr=Inherit: Inherit via internal rule
  Matrix Cross Product : Subsystem
  NB : Constant  Value=sat.NB
  Normalize : Subsystem
  Product : Product  Inputs=5
  Product1 : Product  Multiplication=Matrix(*)
  Product6 : Product  Multiplication=Matrix(*)
  Product7 : Product  Multiplication=Matrix(*)
  Product8 : Product  Inputs=3
  Sum of Elements : Sum  Inputs=+  CollapseMode=Specified dimension  CollapseDim=2
  Sum4 : Sum  Inputs=+-
  Transpose : Math  Operator=transpose
  Vector Concatenate1 : Concatenate  NumInputs=3
  Zero : Constant  Value=0  OutDataTypeStr=Inherit: Inherit via back propagation
  wEarth : Constant  Value=astroConstants.wEarth
  Torque : Outport
  wires:
  r/1 -> Cross Product/2, Air Density/1(r)
  wEarth/1 -> Vector Concatenate1/3
  Zero/1 -> Vector Concatenate1/2, Vector Concatenate1/1
  Vector Concatenate1/1 -> Cross Product/1
  v/1 -> Sum4/1
  Cross Product/1 -> Sum4/2
  Sum4/1 -> Product6/2
  A/1 -> Product6/1
  Product6/1 -> Dot Product3/2, Dot Product3/1, Normalize/1(V)
  Normalize/1(Vnorm) -> Product/2, Transpose/1
  Transpose/1 -> Product7/1
  NB/1 -> Product7/2
  Product7/1 -> Compare To Zero/1, Product8/2
  Constant/1 -> Product8/1
  Compare To Zero/1 -> Product8/3
  Constant1/1 -> Product/1
  Dot Product3/1 -> Product/3
  Air Density/1(rho) -> Product/4
  Cd/1 -> Product/5
  Product8/1 -> Product1/2
  Matrix Cross Product/1(c) -> Sum of Elements/1
  Constant8/1 -> Matrix Cross Product/1(a)
  Product1/1 -> Matrix Cross Product/2(b)
  Sum of Elements/1 -> Torque/1
  Product/1 -> Product1/1

== system eulerEq/DISTURBANCES/Gravity Gradient ==
  I : Inport
  r : Inport  Port=2
  A : Inport  Port=3
  Constant : Constant  Value=3
  Cross Product : vrlib/Utilities/Cross Product
  Divide1 : Product  Inputs=*/
  Dot Product : DotProduct  OutDataTypeStr=Inherit: Inherit via internal rule
  Gain : Gain  Gain=-3*astroConstants.muEarth
  Gain1 : Gain  Gain=-1
  Normalize2 : Subsystem
  Power : Math  Operator=pow
  Product : Product  Multiplication=Matrix(*)
  Product1 : Product
  Sqrt : Sqrt
  Torque : Outport
  wires:
  Product/1 -> Product1/2, Cross Product/2
  Dot Product/1 -> Sqrt/1
  r/1 -> Dot Product/2, Dot Product/1, Normalize2/1(r)
  Sqrt/1 -> Power/1
  Power/1 -> Divide1/2
  Divide1/1 -> Gain/1
  Product1/1 -> Cross Product/1
  Cross Product/1 -> Divide1/1
  Gain1/1 -> Product/2
  A/1 -> Product/1
  Normalize2/1(Out) -> Gain1/1
  Constant/1 -> Power/2
  Gain/1 -> Torque/1
  I/1 -> Product1/1

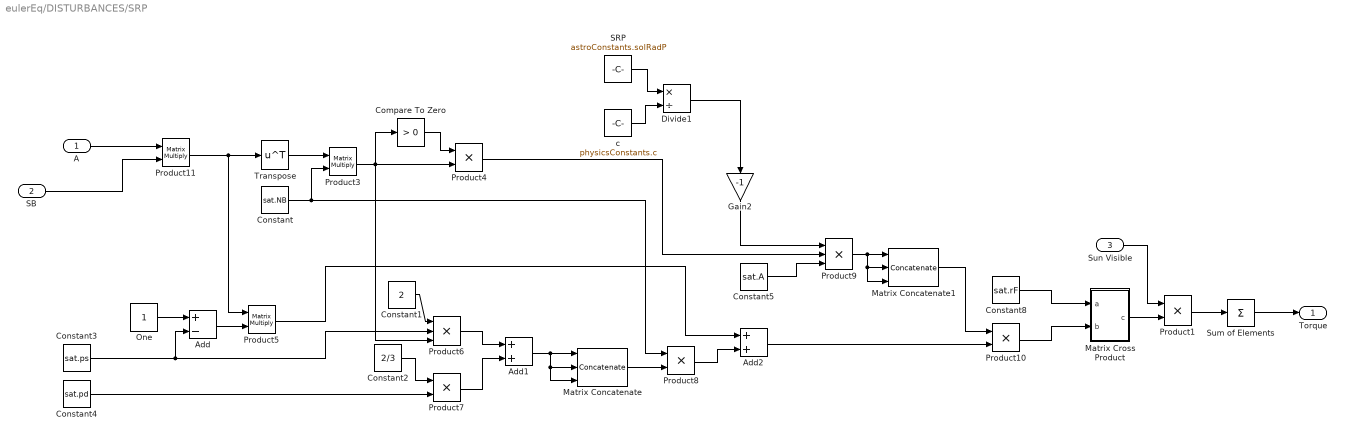
== system eulerEq/DISTURBANCES/SRP ==
  A : Inport
  SB : Inport  Port=2
  Sun Visible : Inport  Port=3
  Add : Sum  Inputs=+-
  Add1 : Sum
  Add2 : Sum
  Compare To Zero : simulink/Logic and Bit Operations/Compare To Zero  relop=>  OutDataTypeStr=boolean
  Constant : Constant  Value=sat.NB
  Constant1 : Constant  Value=2
  Constant2 : Constant  Value=2/3
  Constant3 : Constant  Value=sat.ps  VectorParams1D=off
  Constant4 : Constant  Value=sat.pd  VectorParams1D=off
  Constant5 : Constant  Value=sat.A  VectorParams1D=off
  Constant8 : Constant  Value=sat.rF  VectorParams1D=off
  Divide1 : Product  Inputs=*/
  Gain2 : Gain  Gain=-1
  Matrix Concatenate : Concatenate  NumInputs=3  Mode=Multidimensional array
  Matrix Concatenate1 : Concatenate  NumInputs=3  Mode=Multidimensional array
  Matrix Cross Product : Subsystem
  One : Constant  OutDataTypeStr=Inherit: Inherit via back propagation
  Product{1,4,7..8,10} (5 alike) : Product
  Product11 : Product  Multiplication=Matrix(*)
  Product3 : Product  Multiplication=Matrix(*)
  Product5 : Product  Multiplication=Matrix(*)
  Product6 : Product  Inputs=3
  Product9 : Product  Inputs=3
  SRP : Constant  Value=astroConstants.solRadP
  Sum of Elements : Sum  Inputs=+  CollapseMode=Specified dimension  CollapseDim=2
  Transpose : Math  Operator=transpose
  c : Constant  Value=physicsConstants.c
  Torque : Outport
  wires:
  Constant5/1 -> Product9/3
  Matrix Concatenate/1 -> Product8/2
  c/1 -> Divide1/2
  Add/1 -> Product5/2
  Constant4/1 -> Product7/2
  Product6/1 -> Add1/1
  Product5/1 -> Add2/1
  Product11/1 -> Transpose/1, Product5/1
  Product4/1 -> Product9/2
  SRP/1 -> Divide1/1
  Matrix Concatenate1/1 -> Product10/1
  Add1/1 -> Matrix Concatenate/3, Matrix Concatenate/2, Matrix Concatenate/1
  Constant3/1 -> Product6/2, Add/2
  Constant/1 -> Product8/1, Product3/2
  Product3/1 -> Compare To Zero/1, Product4/2, Product6/3
  Product9/1 -> Matrix Concatenate1/2, Matrix Concatenate1/3, Matrix Concatenate1/1
  Compare To Zero/1 -> Product4/1
  Constant2/1 -> Product7/1
  One/1 -> Add/1
  Product7/1 -> Add1/2
  Gain2/1 -> Product9/1
  Add2/1 -> Product10/2
  Constant1/1 -> Product6/1
  Divide1/1 -> Gain2/1
  Product8/1 -> Add2/2
  Product10/1 -> Matrix Cross Product/2(b)
  Constant8/1 -> Matrix Cross Product/1(a)
  Product1/1 -> Sum of Elements/1
  Matrix Cross Product/1(c) -> Product1/2
  A/1 -> Product11/1
  Sum of Elements/1 -> Torque/1
  Transpose/1 -> Product3/1
  SB/1 -> Product11/2
  Sun Visible/1 -> Product1/1

== system eulerEq/KINEMATICS/312 Matrix ==
  euler Angles : Inport
  Rotation Angles to Direction Cosine Matrix : sharedtransform/Rotation Angles to Direction Cosine Matrix  rotationOrder=ZXY  aMode=aMode
  A : Outport
  wires:
  euler Angles/1 -> Rotation Angles to Direction Cosine Matrix/1
  Rotation Angles to Direction Cosine Matrix/1 -> A/1

== system eulerEq/KINEMATICS/312 Subsystem ==
  w : Inport
  ea : Inport  Port=2
  Enable : EnablePort  StatesWhenEnabling=reset
  Kinematics Euler Angles 312 : Subsystem
  rotmToEul 312 : Subsystem
  dEA : Outport  OutputWhenDisabled=reset  InitialOutput=[0,0,0]
  Aea : Outport  Port=2  OutputWhenDisabled=reset  InitialOutput=zeros(3)
  wires:
  ea/1 -> rotmToEul 312/1(In1), Kinematics Euler Angles 312/1(Euler Angles)
  w/1 -> Kinematics Euler Angles 312/2(Angular Velocity)
  Kinematics Euler Angles 312/1(Euler Angles Dot) -> dEA/1
  rotmToEul 312/1(Out1) -> Aea/1

== system eulerEq/KINEMATICS/312 difEq ==
  w : Inport
  euler Angles : Inport  Port=2
  Cos : Trigonometry  Operator=cos
  Cos1 : Trigonometry  Operator=cos
  Demux : Demux  Outputs=3
  Demux1 : Demux  Outputs=3
  Divide1 : Product  Inputs=*/
  Product{3..6} (4 alike) : Product
  Product7 : Product  Inputs=**/
  Sin : Trigonometry
  Sin1 : Trigonometry
  Sum : Sum  Inputs=|+-
  Sum1 : Sum  Inputs=|++
  Sum3 : Sum  Inputs=|-+
  Terminator : Terminator
  Vector Concatenate : Concatenate  NumInputs=3
  euler Velocities : Outport
  wires:
  Sum3/1 -> Vector Concatenate/3
  Demux1/2 -> Sin1/1, Cos1/1
  Product4/1 -> Sum/2
  Demux/2 -> Sum3/2
  Sin/1 -> Product4/2, Product6/2
  Sin1/1 -> Product7/2
  Demux1/3 -> Sin/1, Cos/1
  Vector Concatenate/1 -> euler Velocities/1
  Product3/1 -> Sum/1
  Demux/1 -> Product4/1, Product5/1
  euler Angles/1 -> Demux1/1
  Product6/1 -> Sum1/2
  Cos/1 -> Product3/2, Product5/2
  Demux/3 -> Product6/1, Product3/1
  Divide1/1 -> Vector Concatenate/1
  Sum1/1 -> Vector Concatenate/2
  Cos1/1 -> Product7/3, Divide1/2
  Product7/1 -> Sum3/1
  w/1 -> Demux/1
  Sum/1 -> Product7/1, Divide1/1
  Product5/1 -> Sum1/1
  Demux1/1 -> Terminator/1

== system eulerEq/KINEMATICS/313 Subsystem ==
  w : Inport
  ea : Inport  Port=2
  Enable : EnablePort  StatesWhenEnabling=reset
  Kinematics Euler Angles 313 : Subsystem
  rotmToEul 313 : Subsystem
  dEA : Outport  OutputWhenDisabled=reset  InitialOutput=[0,0,0]
  Aea : Outport  Port=2  OutputWhenDisabled=reset  InitialOutput=zeros(3)
  wires:
  ea/1 -> Kinematics Euler Angles 313/2(Euler Angles), rotmToEul 313/1(In1)
  rotmToEul 313/1(Out1) -> Aea/1
  Kinematics Euler Angles 313/1(Euler Angles Dot) -> dEA/1
  w/1 -> Kinematics Euler Angles 313/1(Angular Velocity)

== system eulerEq/KINEMATICS/Initial Conditions ==
  reset : Inport
  singularityFlag : Inport  Port=2
  Aea : Inport  Port=3
  AND : Logic  AllPortsSameDT=off  OutDataTypeStr=boolean
  AND1 : Logic  AllPortsSameDT=off  OutDataTypeStr=boolean
  Clock : Clock
  Compare To Zero : simulink/Logic and Bit Operations/Compare To Zero  relop=<=  OutDataTypeStr=boolean
  Constant : Constant  Value=ea0
  In3 : InportShadow
  In4 : InportShadow  Port=2
  Inport1 : InportShadow  Port=3
  NOT : Logic  Operator=NOT  AllPortsSameDT=off  OutDataTypeStr=boolean
  Switch : Switch  Criteria=u2 > Threshold  SaturateOnIntegerOverflow=off  InputSameDT=off
  Switch1 : Switch  Criteria=u2 > Threshold  SaturateOnIntegerOverflow=off  InputSameDT=off
  rotmToEa 312 : Subsystem
  rotmToEa 313 : Subsystem
  ea0 : Outport
  wires:
  singularityFlag/1 -> AND/2
  Switch/1 -> ea0/1
  reset/1 -> AND/1
  Constant/1 -> Switch/1
  Switch1/1 -> Switch/3
  NOT/1 -> AND1/2
  AND/1 -> rotmToEa 312/Enable, Switch1/2
  Clock/1 -> Compare To Zero/1
  AND1/1 -> rotmToEa 313/Enable
  rotmToEa 313/1(ea) -> Switch1/3
  rotmToEa 312/1(ea) -> Switch1/1
  Compare To Zero/1 -> Switch/2
  In3/1 -> AND1/1
  In4/1 -> NOT/1
  Aea/1 -> rotmToEa 312/1(A)
  Inport1/1 -> rotmToEa 313/1(A)

== system eulerEq/KINEMATICS/Singularity Solver ==
  ea : Inport
  AND : Logic  IconShape=distinctive  AllPortsSameDT=off  OutDataTypeStr=boolean
  Abs : Abs  SaturateOnIntegerOverflow=off
  Abs1 : Abs  SaturateOnIntegerOverflow=off
  Compare To Constant : simulink/Logic and Bit Operations/Compare To Constant  relop=>  const=0.1  OutDataTypeStr=boolean
  Compare To Constant1 : simulink/Logic and Bit Operations/Compare To Constant  relop=>  const=0.1  OutDataTypeStr=boolean
  Constant : Constant
  Constant1 : Constant  Value=0
  Previous sample : UnitDelay  InitialCondition=1  SampleTime=-1  HasFrameUpgradeWarning=on
  Selector : Selector  InputPortWidth=3  IndexOptions=Index vector (dialog)  Indices=2  OutputSizes=1
  SinCos : Trigonometry  Operator=sincos
  Switch : Switch  Criteria=u2 > Threshold  SaturateOnIntegerOverflow=off  InputSameDT=off
  Switch1 : Switch  Criteria=u2 > Threshold  SaturateOnIntegerOverflow=off  InputSameDT=off
  Out1 : Outport
  wires:
  ea/1 -> Selector/1
  Compare To Constant/1 -> AND/1
  Compare To Constant1/1 -> Switch1/2, AND/2
  AND/1 -> Switch/2
  Previous sample/1 -> Switch/1
  Switch/1 -> Out1/1, Previous sample/1
  Constant/1 -> Switch1/1
  Switch1/1 -> Switch/3
  Constant1/1 -> Switch1/3
  SinCos/2 -> Abs1/1
  Abs1/1 -> Compare To Constant1/1
  Abs/1 -> Compare To Constant/1
  SinCos/1 -> Abs/1
  Selector/1 -> SinCos/1

== system eulerEq/ORBIT/Earth Orbit ==
  Constant : Constant  Value=earth.r0  VectorParams1D=off
  Constant1 : Constant  Value=3
  Constant2 : Constant  Value=earth.v0  VectorParams1D=off
  Divide1 : Product  Inputs=*/
  Dot Product : DotProduct  OutDataTypeStr=Inherit: Inherit via internal rule
  Gain2 : Gain  Gain=-astroConstants.muSun
  Integrator4 : Integrator  InitialConditionSource=external  InitialCondition=earth.v0
  Integrator5 : Integrator  InitialConditionSource=external  InitialCondition=earth.r0
  Power : Math  Operator=pow
  Sqrt : Sqrt
  r : Outport
  wires:
  Integrator4/1 -> Integrator5/1
  Sqrt/1 -> Power/1
  Gain2/1 -> Divide1/1
  Divide1/1 -> Integrator4/1
  Power/1 -> Divide1/2
  Integrator5/1 -> Gain2/1, r/1, Dot Product/1, Dot Product/2
  Dot Product/1 -> Sqrt/1
  Constant1/1 -> Power/2
  Constant/1 -> Integrator5/2
  Constant2/1 -> Integrator4/2

== system eulerEq/ORBIT/Normalize1 ==
  r : Inport
  Dot Product : DotProduct  OutDataTypeStr=Inherit: Inherit via internal rule
  Product : Product  Inputs=*/
  Sqrt : Sqrt
  Out : Outport
  wires:
  Dot Product/1 -> Sqrt/1
  r/1 -> Dot Product/2, Dot Product/1, Product/1
  Sqrt/1 -> Product/2
  Product/1 -> Out/1

== system eulerEq/ORBIT/Normalize2 ==
  r : Inport
  Dot Product : DotProduct  OutDataTypeStr=Inherit: Inherit via internal rule
  Product : Product  Inputs=*/
  Sqrt : Sqrt
  Out : Outport
  wires:
  Dot Product/1 -> Sqrt/1
  r/1 -> Dot Product/2, Dot Product/1, Product/1
  Sqrt/1 -> Product/2
  Product/1 -> Out/1

== system eulerEq/ORBIT/Normalize3 ==
  r : Inport
  Dot Product : DotProduct  OutDataTypeStr=Inherit: Inherit via internal rule
  Product : Product  Inputs=*/
  Sqrt : Sqrt
  Out : Outport
  wires:
  Dot Product/1 -> Sqrt/1
  r/1 -> Dot Product/2, Dot Product/1, Product/1
  Sqrt/1 -> Product/2
  Product/1 -> Out/1

== system eulerEq/ORBIT/Sat Orbit ==
  Constant1 : Constant  Value=3
  Divide1 : Product  Inputs=*/
  Dot Product : DotProduct  OutDataTypeStr=Inherit: Inherit via internal rule
  Gain2 : Gain  Gain=-astroConstants.muEarth
  Integrator4 : Integrator  InitialCondition=orbit.v0
  Integrator5 : Integrator  InitialCondition=orbit.r0
  Power : Math  Operator=pow
  Sqrt : Sqrt
  r : Outport
  v : Outport  Port=2
  wires:
  Integrator4/1 -> v/1, Integrator5/1
  Sqrt/1 -> Power/1
  Gain2/1 -> Divide1/1
  Divide1/1 -> Integrator4/1
  Power/1 -> Divide1/2
  Integrator5/1 -> Gain2/1, Dot Product/1, Dot Product/2, r/1
  Dot Product/1 -> Sqrt/1
  Constant1/1 -> Power/2

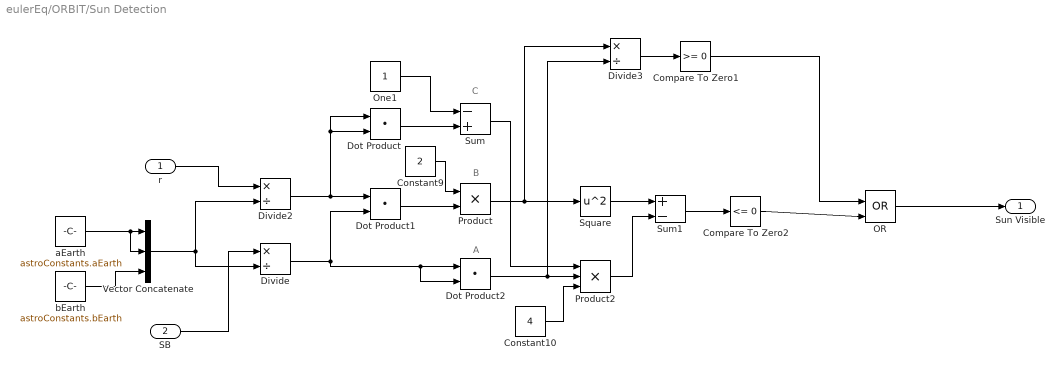
== system eulerEq/ORBIT/Sun Detection ==
  note: C
  note: B
  note: A
  r : Inport
  SB : Inport  Port=2
  Compare To Zero1 : simulink/Logic and Bit Operations/Compare To Zero  relop=>=  OutDataTypeStr=boolean
  Compare To Zero2 : simulink/Logic and Bit Operations/Compare To Zero  relop=<=  OutDataTypeStr=boolean
  Constant10 : Constant  Value=4
  Constant9 : Constant  Value=2
  Divide : Product  Inputs=*/
  Divide2 : Product  Inputs=*/
  Divide3 : Product  Inputs=*/
  Dot Product : DotProduct  OutDataTypeStr=Inherit: Inherit via internal rule
  Dot Product1 : DotProduct  OutDataTypeStr=Inherit: Inherit via internal rule
  Dot Product2 : DotProduct  OutDataTypeStr=Inherit: Inherit via internal rule
  OR : Logic  Operator=OR  IconShape=distinctive  AllPortsSameDT=off  OutDataTypeStr=boolean
  One1 : Constant  OutDataTypeStr=Inherit: Inherit via back propagation
  Product : Product
  Product2 : Product  Inputs=3
  Square : Math  Operator=square
  Sum : Sum  Inputs=-+
  Sum1 : Sum  Inputs=+-
  Vector Concatenate : Concatenate  NumInputs=3
  aEarth : Constant  Value=astroConstants.aEarth
  bEarth : Constant  Value=astroConstants.bEarth
  Sun Visible : Outport
  wires:
  Divide3/1 -> Compare To Zero1/1
  OR/1 -> Sun Visible/1
  Compare To Zero2/1 -> OR/2
  Square/1 -> Sum1/1
  One1/1 -> Sum/1
  aEarth/1 -> Vector Concatenate/2, Vector Concatenate/1
  Constant9/1 -> Product/1
  Dot Product1/1 -> Product/2
  Divide/1 -> Dot Product2/1, Dot Product2/2, Dot Product1/2
  Product/1 -> Divide3/1, Square/1
  Sum1/1 -> Compare To Zero2/1
  Dot Product2/1 -> Divide3/2, Product2/2
  r/1 -> Divide2/1
  Sum/1 -> Product2/1
  Constant10/1 -> Product2/3
  Divide2/1 -> Dot Product1/1, Dot Product/2, Dot Product/1
  Product2/1 -> Sum1/2
  Vector Concatenate/1 -> Divide2/2, Divide/2
  Dot Product/1 -> Sum/2
  SB/1 -> Divide/1
  bEarth/1 -> Vector Concatenate/3
  Compare To Zero1/1 -> OR/1

== system eulerEq/ATTITUDE DETERMINATION/Subsystem/Normalize ==
  r : Inport
  Dot Product : DotProduct  OutDataTypeStr=Inherit: Inherit via internal rule
  Product : Product  Inputs=*/
  Sqrt : Sqrt
  Out : Outport
  wires:
  Dot Product/1 -> Sqrt/1
  r/1 -> Dot Product/2, Dot Product/1, Product/1
  Sqrt/1 -> Product/2
  Product/1 -> Out/1

== system eulerEq/ATTITUDE DETERMINATION/Subsystem/Normalize1 ==
  r : Inport
  Dot Product : DotProduct  OutDataTypeStr=Inherit: Inherit via internal rule
  Product : Product  Inputs=*/
  Sqrt : Sqrt
  Out : Outport
  wires:
  Dot Product/1 -> Sqrt/1
  r/1 -> Dot Product/2, Dot Product/1, Product/1
  Sqrt/1 -> Product/2
  Product/1 -> Out/1

== system eulerEq/CONTROL/BDOT SPIN RATE DAMPING /CROSS MATRIX ==
  Measured w : Inport
  Constant : Constant  Value=0
  Gain : Gain  Gain=-1
  Matrix Concatenate : Concatenate  NumInputs=3  Mode=Multidimensional array  ConcatenateDimension=2
  Selector : Selector  InputPortWidth=7  IndexOptions=Index vector (dialog)  Indices=[7 6 2]  OutputSizes=1
  Selector1 : Selector  InputPortWidth=7  IndexOptions=Index vector (dialog)  Indices=[3 7 4]  OutputSizes=1
  Selector2 : Selector  InputPortWidth=7  IndexOptions=Index vector (dialog)  Indices=[5 1 7]  OutputSizes=1
  Transpose : Math  Operator=transpose
  Vector Concatenate : Concatenate  NumInputs=3
  w^ : Outport
  wires:
  Measured w/1 -> Gain/1, Vector Concatenate/1
  Constant/1 -> Vector Concatenate/3
  Vector Concatenate/1 -> Selector/1, Selector1/1, Selector2/1
  Selector1/1 -> Matrix Concatenate/2
  Selector/1 -> Matrix Concatenate/1
  Selector2/1 -> Matrix Concatenate/3
  Gain/1 -> Vector Concatenate/2
  Matrix Concatenate/1 -> Transpose/1
  Transpose/1 -> w^/1

== system eulerEq/CONTROL/POINTING ERROR/POINTING ERROR (DEG) ==
  A * Ad^T : Inport
  Acos : Trigonometry  Operator=acos
  Add1 : Sum  Inputs=+
  Constant1 : Constant
  Constant2 : Constant  Value=2
  Divide : Product  Inputs=*/
  Extract Diagonal : matrix_library/Extract Diagonal
      settings: LibrarySourceBlock=|
      | simulink/Matrix
      | Operations/Extract Diagonal
  Radians to Degrees : simulink_extras/Transformations/Radians to Degrees
  Subtract : Sum  Inputs=+-
  Degrees out : Outport
  wires:
  Radians to Degrees/1 -> Degrees out/1
  Subtract/1 -> Divide/1
  Add1/1 -> Subtract/1
  Constant2/1 -> Divide/2
  Divide/1 -> Acos/1
  Extract Diagonal/1 -> Add1/1
  Constant1/1 -> Subtract/2
  A * Ad^T/1 -> Extract Diagonal/1
  Acos/1 -> Radians to Degrees/1
